simulink model "turbines2tune"  (R2025b)
settings: Solver=FixedStepAuto  StartTime=0.0  StopTime=200  FixedStep=Ts_outer  RelTol=1e-3
InitFcn:
  | turbine_model_constants;
values from neighbouring files (symbols this model uses):
  A = Simulink.Parameter(R.Value^2*pi)    [turbine_constants_from_yaml.m]    (also in turbine_model_constants.m)
  beta_opt_vector = Simulink.Parameter(beta_array)    [turbine_constants_from_yaml.m]    (also in turbine_model_constants.m)
  beta_vector = tables{4}    [gen_xref_ref.m]    (also in get_look_up_tables.m = zeros(1, 20); turbine_constants_from_yaml.m = Simulink.Parameter(tables{4}); turbine_model_constants.m = Simulink.Parameter(tables{4}))
  c_beta_dot = Simulink.Parameter(0.5)    [turbine_constants_from_yaml.m]    (also in turbine_model_constants.m = Simulink.Parameter(0.1))
  c_gamma_dot = Simulink.Parameter(0.5*pi/180)    [turbine_constants_from_yaml.m]    (also in turbine_model_constants.m = Simulink.Parameter(1/180*pi))
  cp_max = Simulink.Parameter(max(cp_table.Value(:))*0.99)    [turbine_constants_from_yaml.m]    (also in turbine_model_constants.m)
  cp_opt_keys = Simulink.Parameter(cell2mat(cp_vector))    [turbine_constants_from_yaml.m]    (also in turbine_model_constants.m)
  cp_table = tables{1}    [gen_xref_ref.m]    (also in get_look_up_tables.m = zeros(20, 20); turbine_constants_from_yaml.m = Simulink.Parameter(tables{1}); turbine_model_constants.m = Simulink.Parameter(tables{1}))
  ct_table = tables{2}    [gen_xref_ref.m]    (also in get_look_up_tables.m = zeros(20, 20); turbine_constants_from_yaml.m = Simulink.Parameter(tables{2}); turbine_model_constants.m = Simulink.Parameter(tables{2}))
  JT = Simulink.Parameter(10^9)    [turbine_constants_from_yaml.m]    (also in turbine_model_constants.m = Simulink.Parameter(2.052*10^8*3))
  lambda_opt_vector = Simulink.Parameter(lambda_array)    [turbine_constants_from_yaml.m]    (also in turbine_model_constants.m)
  lambda_vector = tables{5}    [gen_xref_ref.m]    (also in turbine_constants_from_yaml.m = Simulink.Parameter(tables{5}); turbine_model_constants.m = Simulink.Parameter(tables{5}))
  mu = Simulink.Parameter(0.95)    [turbine_constants_from_yaml.m]    (also in turbine_model_constants.m)
  Nt = Simulink.Parameter(10)    [turbine_constants_from_yaml.m]    (also in turbine_model_constants.m)
  omega_safety_increase = Simulink.Parameter(1.0)    [turbine_constants_from_yaml.m]    (also in turbine_model_constants.m = Simulink.Parameter(1.02))
  P_omega_dot = Simulink.Parameter(0.01)    [turbine_constants_from_yaml.m]    (also in turbine_model_constants.m = Simulink.Parameter(0.5))
  P_omega_dot_negative = Simulink.Parameter(0.05)    [turbine_model_constants.m]
  R = Simulink.Parameter(80)    [turbine_constants_from_yaml.m]    (also in turbine_model_constants.m = Simulink.Parameter(142); visualise.m = linspace(0.2, 0.7, nColors)')
  rho = Simulink.Parameter(1.225)    [turbine_constants_from_yaml.m]    (also in turbine_model_constants.m)
  Ts = Simulink.Parameter(1)    [turbine_constants_from_yaml.m]    (also in turbine_model_constants.m = Simulink.Parameter(0.1))
  Ts_inner = Simulink.Parameter(1)    [turbine_model_constants.m]
  x0 = Simulink.Parameter([0,0,0])    [turbine_constants_from_yaml.m]    (also in turbine_model_constants.m)
undefined symbols (not defined in the file or in its folder): DiscIntNeverNeededParam, f
libraries: instrumentlib x3, simulink_extras x1
settings Model: Creator=kohlh  LastModifiedBy=akohlheb

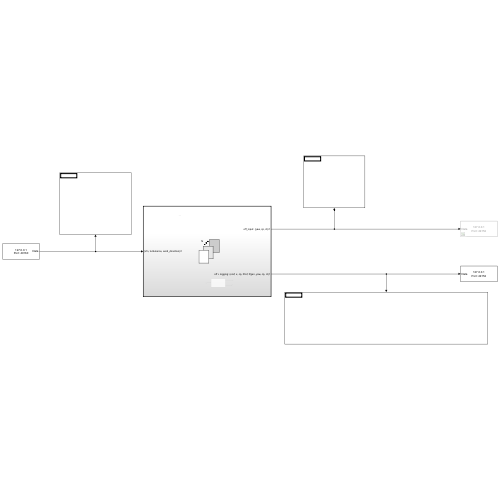
[thumbnail: Simulink's stored preview of the top-level diagram]
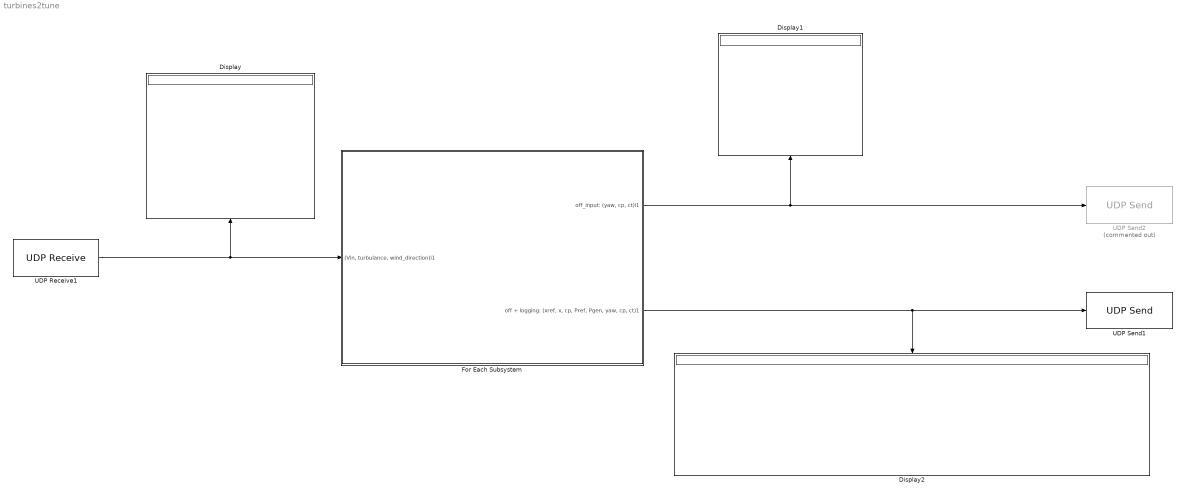
== system turbines2tune ==
  Display : Display
  Display1 : Display
  Display2 : Display
  For Each Subsystem : Subsystem  TreatAsAtomicUnit=on
  UDP Receive1 : instrumentlib/UDP Receive  LocalAddress=127.0.0.1  LocalPort=49160  EnablePortSharing=off  Host=127.0.0.1  Port=49152  GetLatestData=off  DataSize=[Nt,3]  DataType=double  ASCIIFormatting=%f,  Terminator=LF  CustomTerminator=10  ByteOrder=big-endian  EnableBlockingMode=on  Timeout=30  SampleTime=Ts  SimulateUsing=Interpreted execution
  UDP Send1 : instrumentlib/UDP Send  Host=127.0.0.1  Port=49152  LocalAddress=127.0.0.1  LocalPort=49160  EnablePortSharing=off  OutputDatagramPacketSize=512*12*Nt  ByteOrder=big-endian  EnableBlockingMode=on  SimulateUsing=Interpreted execution
  UDP Send2 : instrumentlib/UDP Send  Commented=on  Host=127.0.0.1  Port=49152  LocalAddress=127.0.0.1  LocalPort=49160  EnablePortSharing=off  OutputDatagramPacketSize=512*3*Nt  ByteOrder=big-endian  EnableBlockingMode=on  SimulateUsing=Interpreted execution
  wires:
  UDP Receive1/1 -> For Each Subsystem/1("(Vin, turbulance, wind_direction)i1"), Display/1
  For Each Subsystem/2("off + logging: (xref, x, cp, Pref, Pgen, yaw, cp, ct)1") -> UDP Send1/1, Display2/1
  For Each Subsystem/1("off_input: (yaw, cp, ct)i1") -> Display1/1, UDP Send2/1

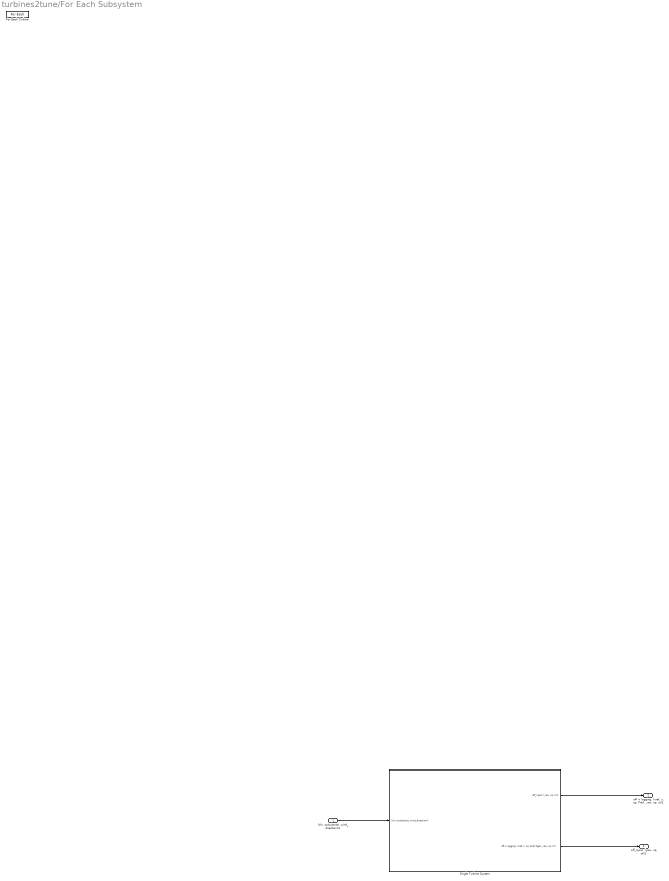
== system turbines2tune/For Each Subsystem ==
  "(Vin, turbulance, wind_direction)i1" : Inport  Partition=on  PartitionDimension=1  PartitionWidth=1  PartitionOffset=0
  For Each Turbine : ForEach  DisableCoverage=on
  Single Turbine System : Subsystem
  "off_input: (yaw, cp, ct)i1" : Outport  ConcatenationDimension=1
  "off + logging: (xref, x, cp, Pref, Pgen, yaw, cp, ct)1" : Outport  Port=2  ConcatenationDimension=1
  wires:
  "(Vin, turbulance, wind_direction)i1"/1 -> Single Turbine System/1("(Vin, turbulance, wind_direction)i")
  Single Turbine System/2("off + logging: (xref, x, cp, Pref, Pgen, yaw, cp, ct)") -> "off_input: (yaw, cp, ct)i1"/1
  Single Turbine System/1("off_input: (yaw, cp, ct)i") -> "off + logging: (xref, x, cp, Pref, Pgen, yaw, cp, ct)1"/1

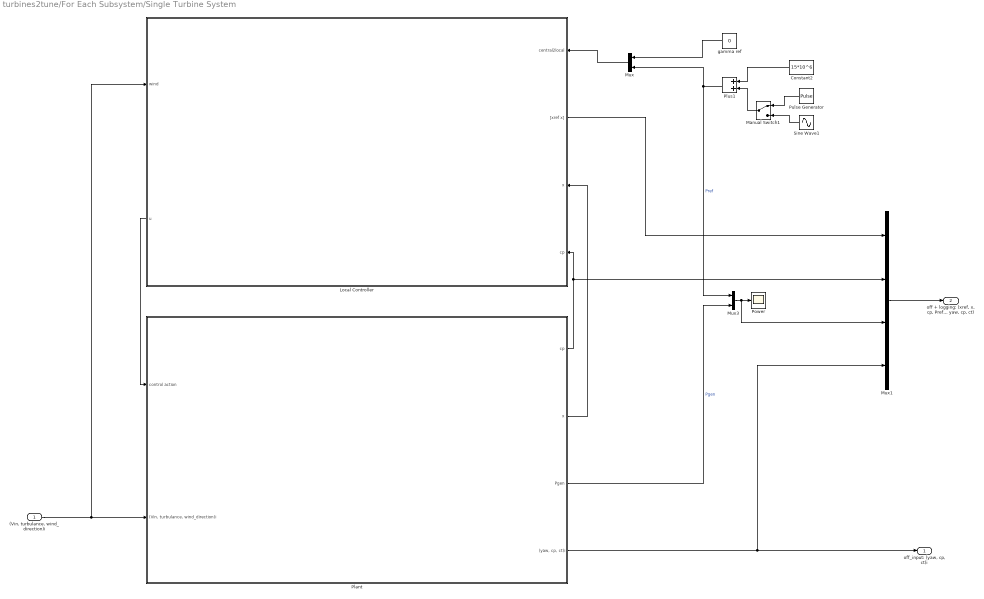
== system turbines2tune/For Each Subsystem/Single Turbine System ==
  "(Vin, turbulance, wind_direction)i" : Inport
  Constant2 : Constant  Value=15*10^6
  Local Controller : Subsystem
      settings: PortSchema="{\"entries\":[{\"content\":{\"sides\":[{\"content\":{\"connectorIds\":[\"In1\",\"Out2\",\"In2\",\"In3\"]},\"type\":\"ConnectorPlacement.EquallySpacedRectSide\",\"uuid\":\"1274bf49-ceae-40b5-8168-864c275c8277\"},{\"content\":{\"connectorIds\":[\"In4\",\"Out1\"],\"side\":\"RIGHT\"},\"type\":\"ConnectorPlacement.EquallySpacedRectSide\",\"uuid\":\"983d855e-2fb7-4029-8a1e-74d0395d6e6b\"},{\"content\":{\"side\":\"TOP\"},\"type\":\"ConnectorPlacement.EquallySpacedRectSide\",\"uuid\":\"78e40a3c-46aa-4158-bc61-97e5b88f823b\"},{\"content\":{\"side\":\"BOTTOM\"},\"type\":\"ConnectorPlacement.EquallySpacedRectSide\",\"uuid\":\"db79cd87-5583-4254-9385-067380eca232\"}]},\"type\":\"ConnectorPlacement.EquallySpacedConnector\",\"uuid\":\"902a270f-1fdc-458f-b9eb-4015978e6616\"}],\"packageUris\":[\"http://schema.mathworks.com/mf0/Connector/R2020b\"],\"version\":\"1.0\"}"
  Manual Switch1 : ManualSwitch
  Mux : Mux  Inputs=2
  Mux1 : Mux
  Mux3 : Mux  Inputs=2
  Plant : Subsystem
  Plus1 : Sum
  Power : Scope
      settings: ActiveDisplayYMinimum=-2.5E+6  ActiveDisplayYMaximum=2.2500000000000004E+7  DataLoggingVariableName=ScopeData2
  Pulse Generator : DiscretePulseGenerator  PulseType=Time based  Amplitude=5*10^6  Period=4000  PulseWidth=50
  Sine Wave1 : Sin  Amplitude=5*10^6  Frequency=3.24/1000  SampleTime=0
  gamma ref : Constant  Value=0
  "off_input: (yaw, cp, ct)i" : Outport
  "off + logging: (xref, x, cp, Pref, Pgen, yaw, cp, ct)" : Outport  Port=2
  wires:
  Local Controller/2("[xref x]") -> Mux1/1
  Plus1/1 -> Mux/2, Mux3/1  "Pref"
  Constant2/1 -> Plus1/1
  Manual Switch1/1 -> Plus1/2
  Mux/1 -> Local Controller/1(central2local)
  Pulse Generator/1 -> Manual Switch1/1
  Plant/3(Pgen) -> Mux3/2  "Pgen"
  "(Vin, turbulance, wind_direction)i"/1 -> Local Controller/4(wind), Plant/2("(Vin, turbulance, wind_direction)i")
  Mux1/1 -> "off + logging: (xref, x, cp, Pref, Pgen, yaw, cp, ct)"/1
  Sine Wave1/1 -> Manual Switch1/2
  Local Controller/1(u) -> Plant/1(control action)
  Plant/4("(yaw, cp, ct)i") -> Mux1/4, "off_input: (yaw, cp, ct)i"/1
  Plant/1(cp) -> Local Controller/3(cp), Mux1/2
  Plant/2(x) -> Local Controller/2(x)
  Mux3/1 -> Mux1/3, Power/1
  gamma ref/1 -> Mux/1

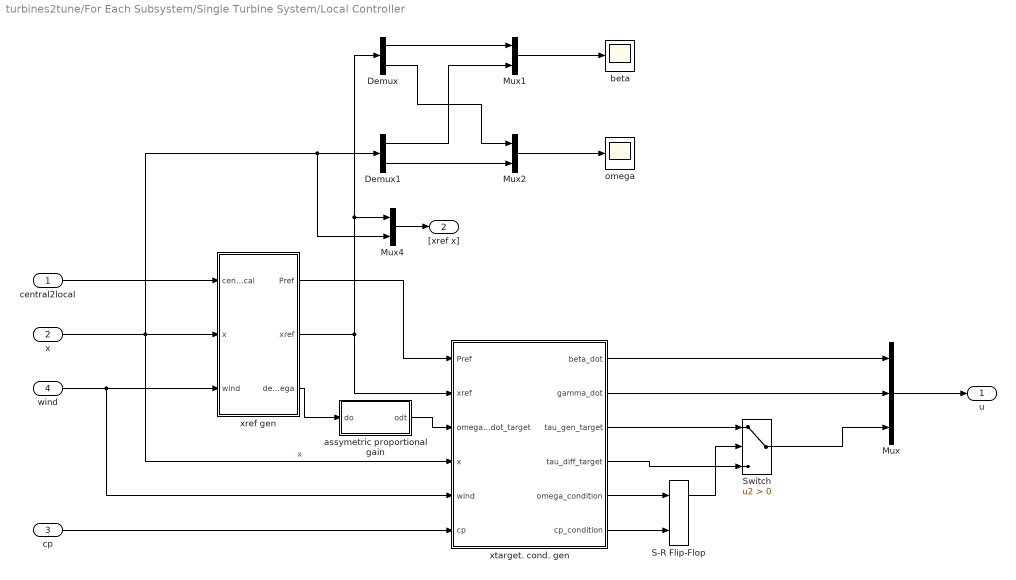
== system turbines2tune/For Each Subsystem/Single Turbine System/Local Controller ==
  central2local : Inport
  x : Inport  Port=2
  cp : Inport  Port=3
  wind : Inport  Port=4
  Demux : Demux  Outputs=3
  Demux1 : Demux  Outputs=3
  Mux : Mux  Inputs=3
  Mux1 : Mux  Inputs=2
  Mux2 : Mux  Inputs=2
  Mux4 : Mux  Inputs=2
  S-R Flip-Flop : simulink_extras/Flip Flops/S-R Flip-Flop  initial_condition=0
  Switch : Switch  Criteria=u2 > Threshold  SaturateOnIntegerOverflow=off  InputSameDT=off
  assymetric proportional gain : MATLAB Function  TreatAsAtomicUnit=on
  beta : Scope
      settings: ActiveDisplayYMinimum=-2.9999999999999991  ActiveDisplayYMaximum=27
  omega : Scope
      settings: ActiveDisplayYMinimum=-0.25747285201612957  ActiveDisplayYMaximum=2.3172556681451666
  xref gen : MATLAB Function  TreatAsAtomicUnit=on
  xtarget. cond. gen : MATLAB Function  TreatAsAtomicUnit=on
  u : Outport
  "[xref x]" : Outport  Port=2
  wires:
  central2local/1 -> xref gen/1(central2local)
  xref gen/2(xref) -> Mux4/1, Demux/1, xtarget. cond. gen/2(xref)
  Mux/1 -> u/1
  xtarget. cond. gen/1(beta_dot) -> Mux/1
  xtarget. cond. gen/2(gamma_dot) -> Mux/2
  xtarget. cond. gen/3(tau_gen_target) -> Switch/1
  xtarget. cond. gen/4(tau_diff_target) -> Switch/3
  xtarget. cond. gen/6(cp_condition) -> S-R Flip-Flop/2
  x/1 -> xtarget. cond. gen/4(x), Mux4/2, Demux1/1, xref gen/2(x)  "x"
  wind/1 -> xtarget. cond. gen/5(wind), xref gen/3(wind)
  Switch/1 -> Mux/3
  S-R Flip-Flop/1 -> Switch/2
  xtarget. cond. gen/5(omega_condition) -> S-R Flip-Flop/1
  cp/1 -> xtarget. cond. gen/6(cp)
  xref gen/3(delta_omega) -> assymetric proportional gain/1(do)
  xref gen/1(Pref) -> xtarget. cond. gen/1(Pref)
  Mux1/1 -> beta/1
  Mux2/1 -> omega/1
  Demux/1 -> Mux1/1
  Demux1/3 -> Mux2/2
  Demux1/1 -> Mux1/2
  Demux/3 -> Mux2/1
  Mux4/1 -> "[xref x]"/1
  assymetric proportional gain/1(odt) -> xtarget. cond. gen/3(omega_dot_target)

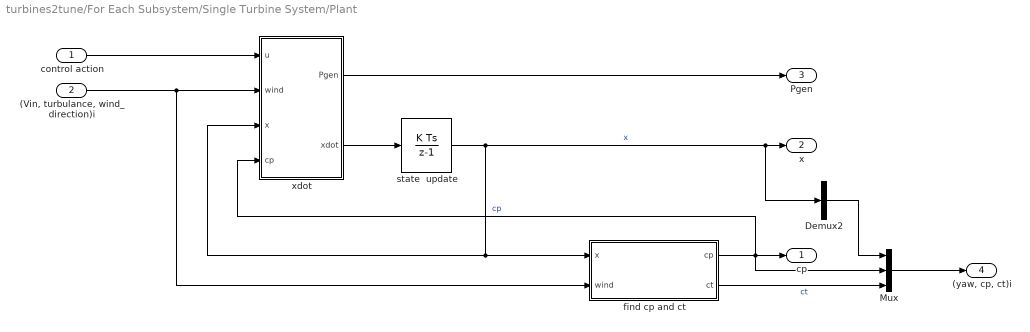
== system turbines2tune/For Each Subsystem/Single Turbine System/Plant ==
  control action : Inport
  "(Vin, turbulance, wind_direction)i" : Inport  Port=2
  Demux2 : Demux  Outputs=3
  Mux : Mux  Inputs=3
  find cp and ct : MATLAB Function  TreatAsAtomicUnit=on
  state  update : DiscreteIntegrator  InitialCondition=x0  SampleTime=-1  LimitOutput=on  ICPrevOutput=DiscIntNeverNeededParam  ICPrevScaledInput=DiscIntNeverNeededParam
  xdot : MATLAB Function  TreatAsAtomicUnit=on
  cp : Outport
  x : Outport  Port=2
  Pgen : Outport  Port=3
  "(yaw, cp, ct)i" : Outport  Port=4
  wires:
  "(Vin, turbulance, wind_direction)i"/1 -> find cp and ct/2(wind), xdot/2(wind)
  xdot/2(xdot) -> state  update/1
  state  update/1 -> Demux2/1, x/1, find cp and ct/1(x), xdot/3(x)  "x"
  control action/1 -> xdot/1(u)
  xdot/1(Pgen) -> Pgen/1
  find cp and ct/1(cp) -> Mux/2, cp/1, xdot/4(cp)  "cp"
  find cp and ct/2(ct) -> Mux/3  "ct"
  Demux2/2 -> Mux/1
  Mux/1 -> "(yaw, cp, ct)i"/1

== matlab function turbines2tune/For Each Subsystem/Single Turbine System/Plant/xdot ==
  data: Pgen output; u input; xdot output; wind input; x input; cp input; JT parameter; A parameter; rho parameter; mu parameter
function [Pgen, xdot] = fcn(u, wind, x, cp, JT, A, rho, mu)

Vin = wind(1);
turbulance = 1-wind(2);
wind_direction = wind(3);

beta_dot = u(1);
gamma_dot = u(2);
tau_gen = u(3);

gamma = x(2);
omega = x(3);

%eliminating division by 0
if omega < 0.1 && omega >= 0
    omega = 0.1;
    tau_gen = 0;
    % if there is no motion backwards acc due to tau aero is not allowed
    tau_aero = max(0, cp * Vin^3 * rho * A * 1/2 * turbulance * cos(wind_direction-gamma)^3 / omega);
elseif omega < 0
    tau_aero = abs(cp * Vin^3 * rho * A * 1/2 * turbulance * cos(wind_direction-gamma)^3 / omega);
    tau_gen = 0;
else
    tau_aero = cp * Vin^3 * rho * A * 1/2 * turbulance * cos(wind_direction-gamma)^3 / omega;
end

omega_dot = (tau_aero - tau_gen)/JT;

xdot = [beta_dot, gamma_dot, omega_dot];
Pgen = tau_gen * omega * mu;

end

== matlab function turbines2tune/For Each Subsystem/Single Turbine System/Local Controller/assymetric proportional gain ==
  data: do input; odt output; P_omega_dot parameter; P_omega_dot_negative parameter
function odt = P(do, P_omega_dot, P_omega_dot_negative)
if do > 0
    odt = P_omega_dot * do;
else
    odt = P_omega_dot_negative * do;
end

== matlab function turbines2tune/For Each Subsystem/Single Turbine System/Local Controller/xref gen ==
  data: central2local input; Pref output; x input; wind input; xref output; mu parameter; lambda_vector parameter; beta_vector parameter; cp_table parameter; R parameter; rho parameter; A parameter; cp_max parameter; delta_omega output; cp_opt_keys parameter; beta_opt_vector parameter; c_beta_dot parameter; Ts_inner parameter; lambda_opt_vector parameter
function [Pref, xref, delta_omega] = xrefgen(central2local,  x, wind, mu, lambda_vector, beta_vector, cp_table, R, rho, A, cp_max, cp_opt_keys, beta_opt_vector, c_beta_dot, Ts_inner, lambda_opt_vector)
    Vin = wind(1);
    turbulance = 1-wind(2);
    wind_direction = wind(3);

    Pref = central2local(2);
    gamma_ref = wind_direction; %central2local(1);
    
    beta = x(1);
    gamma = x(2);
    omega = x(3);
    
    %cap cpref to avoid oscillation at the boundary
    Pref = max(min(Pref, (1/2 * Vin^3 * rho * A * mu * turbulance*cos(wind_direction - gamma)^3)*cp_max),0);
    if cos(wind_direction - gamma) > 0
        cpref = Pref/(1/2 * Vin^3 * rho * A * mu * turbulance*cos(wind_direction - gamma)^3);
    else
        cpref = 0;
    end

    
    %find closest cp opt key that is larger than cpref
    [closest_cp, ~] = min(abs((cp_opt_keys >= cpref) - cpref));
    [~,closest_cp_index] = min(abs(cp_opt_keys - closest_cp));
    beta_opt = beta_opt_vector(closest_cp_index);
    %find beta that is achieveable with delta beta due to descrete steps
    deltabeta = c_beta_dot * Ts_inner;
    beta_over = ceil((beta_opt - beta)/deltabeta) * deltabeta + beta;
    beta_under = floor((beta_opt - beta)/deltabeta) * deltabeta + beta;

    beta_ref = beta_under;

    cp_at_beta_opt = NaN;
    for i = 1:length(beta_vector)-1
        if beta_vector(i) <= beta_ref && beta_vector(i+1) >= beta_ref
            cp_at_beta_opt = cp_table(1:end,i) * abs((beta_ref - beta_vector(i+1))/(beta_vector(i+1) - beta_vector(i))) + cp_table(1:end,i+1) * abs((beta_ref - beta_vector(i))/(beta_vector(i+1) - beta_vector(i)));
            break
        end
    end

    lambda_ref = NaN;
    for i = 1:length(beta_vector)-1
        if (cp_at_beta_opt(i) <= cpref && cp_at_beta_opt(i+1) >= cpref) || (cp_at_beta_opt(i+1) <= cpref && cp_at_beta_opt(i) >= cpref)
            lambda_ref = lambda_vector(i) * abs((cpref - cp_at_beta_opt(i+1))/(cp_at_beta_opt(i+1) - cp_at_beta_opt(i))) + lambda_vector(i+1) * abs((cpref - cp_at_beta_opt(i))/(cp_at_beta_opt(i+1) - cp_at_beta_opt(i)));
            break
        end
    end

    if isnan(lambda_ref)
        beta_ref = beta_over;

        for i = 1:length(beta_vector)-1
            if beta_vector(i) <= beta_ref && beta_vector(i+1) >= beta_ref
                cp_at_beta_opt = cp_table(1:end,i) * abs((beta_ref - beta_vector(i+1))/(beta_vector(i+1) - beta_vector(i))) + cp_table(1:end,i+1) * abs((beta_ref - beta_vector(i))/(beta_vector(i+1) - beta_vector(i)));
                break
            end
        end

        for i = 1:length(beta_vector)-1
            if (cp_at_beta_opt(i) <= cpref && cp_at_beta_opt(i+1) >= cpref) || (cp_at_beta_opt(i+1) <= cpref && cp_at_beta_opt(i) >= cpref)
                lambda_ref = lambda_vector(i) * abs((cpref - cp_at_beta_opt(i+1))/(cp_at_beta_opt(i+1) - cp_at_beta_opt(i))) + lambda_vector(i+1) * abs((cpref - cp_at_beta_opt(i))/(cp_at_beta_opt(i+1) - cp_at_beta_opt(i)));
                break
            end
        end
    end
    if isnan(lambda_ref)
        beta_ref = beta_opt;
        for i = 1:length(beta_vector)-1
            if beta_vector(i) <= beta_ref && beta_vector(i+1) >= beta_ref
                cp_at_beta_opt = cp_table(1:end,i) * abs((beta_ref - beta_vector(i+1))/(beta_vector(i+1) - beta_vector(i))) + cp_table(1:end,i+1) * abs((beta_ref - beta_vector(i))/(beta_vector(i+1) - beta_vector(i)));
                break
            end
        end

        for i = 1:length(beta_vector)-1
            if (cp_at_beta_opt(i) <= cpref && cp_at_beta_opt(i+1) >= cpref) || (cp_at_beta_opt(i+1) <= cpref && cp_at_beta_opt(i) >= cpref)
                lambda_ref = lambda_vector(i) * abs((cpref - cp_at_beta_opt(i+1))/(cp_at_beta_opt(i+1) - cp_at_beta_opt(i))) + lambda_vector(i+1) * abs((cpref - cp_at_beta_opt(i))/(cp_at_beta_opt(i+1) - cp_at_beta_opt(i)));
                break
            end
        end
    end
    if isnan(lambda_ref)
        lambda_ref = lambda_opt_vector(closest_cp_index);
    end
    
    omega_ref = lambda_ref * Vin * cos(wind_direction - gamma) / R;   
    xref = [beta_ref, gamma_ref, omega_ref];
    delta_omega = (omega_ref - omega)/omega_ref;
end

== matlab function turbines2tune/For Each Subsystem/Single Turbine System/Local Controller/xtarget. cond. gen ==
  data: Pref input; xref input; omega_dot_target input; beta_dot output; gamma_dot output; tau_gen_target output; tau_diff_target output; omega_condition output; x input; wind input; cp input; R parameter; lambda_vector parameter; beta_vector parameter; cp_table parameter; mu parameter; rho parameter; A parameter; omega_safety_increase parameter; cp_condition output; Ts_inner parameter; c_beta_dot parameter; c_gamma_dot parameter; JT parameter
function [beta_dot, gamma_dot, tau_gen_target, tau_diff_target, omega_condition, cp_condition] = tg(Pref, xref,omega_dot_target, x, wind, cp, R, lambda_vector, beta_vector, cp_table, mu, rho, A, omega_safety_increase, Ts_inner, c_beta_dot, c_gamma_dot, JT)
beta = x(1);
gamma = x(2);
omega = x(3);

Vin = wind(1);
turbulance = 1-wind(2);
wind_direction = wind(3);

betaref = xref(1);
gammaref = xref(2);
omegaref = xref(3);

lambda = omega * R / (Vin * cos(wind_direction - gamma));

lambda_index_under = 0;
for i=1:length(lambda_vector)-1
    if lambda>lambda_vector(i)
        lambda_index_under = i;
    end
end

if lambda_index_under == 0
    lambda_under_coef = 1;
    lambda_index_under = 1;
elseif lambda > lambda_vector(end)
    lambda_under_coef = 0;
else
    lambda_under_coef = abs((lambda_vector(lambda_index_under+1) - lambda)/(lambda_vector(lambda_index_under) - lambda_vector(lambda_index_under+1)));
end

cp_at_omega = cp_table(lambda_index_under, 1:end) * lambda_under_coef +  cp_table(lambda_index_under+1, 1:end) * (1-lambda_under_coef);

if omega <= 0
    tau_gen_target = 0;
else
    tau_gen_target = Pref/(omega*mu);
end
if isnan(tau_gen_target)
    tau_gen_target = 0;
end

tau_aero_target = JT * omega_dot_target + tau_gen_target; % to reach omega dot target
if cos(wind_direction - gamma) > 0
    if omega > 0
        cp_target = tau_aero_target* omega / (1/2 * rho * A * Vin^3 * turbulance * cos(wind_direction - gamma)^3);
    elseif omega == 0
        cp_target = 0.5;
    else
        cp_target = -tau_aero_target* omega / (1/2 * rho * A * Vin^3 * turbulance * cos(wind_direction - gamma)^3);
    end
else
    cp_target = 0;
end

cpmin = abs(tau_gen_target * omega / (1/2 * rho * A * Vin^3 * turbulance * cos(wind_direction - gamma)^3));

cp_increase_direction = 1;
cp_target = max(0, cp_target);
if cp_target > max(cp_at_omega)
    [~, beta_upper_index] = max(cp_at_omega);
    beta_target_online = beta_vector(beta_upper_index);
else
    beta_target_online = nan;
    for i=length(beta_vector):-1:2 % going from higher beta valeus
        if (cp_at_omega(i-1) >= cp_target && cp_at_omega(i) <= cp_target) || (cp_at_omega(i) >= cp_target && cp_at_omega(i-1) <= cp_target)
            beta_target_upper_index = i;
            beta_upper_coef = abs((cp_at_omega(beta_target_upper_index-1)- cp_target)/(cp_at_omega(beta_target_upper_index-1) - cp_at_omega(beta_target_upper_index)));
            beta_target_online = beta_vector(beta_target_upper_index) * beta_upper_coef + beta_vector(beta_target_upper_index-1) * (1-beta_upper_coef);
            if cp_at_omega(i-1) <= cp_at_omega(i)
                cp_increase_direction = 1;
            else
                cp_increase_direction = -1;
            end
            break
        end
    end
end

beta_target = beta_target_online;

if abs(beta_target - beta) > Ts_inner * c_beta_dot
    if beta_target > beta
        beta_dot = c_beta_dot;
    else
        beta_dot = -c_beta_dot;
    end
else
    if abs(omega_dot_target) > 10^(-5)
        if omega_dot_target > 0
            if beta_target > beta
                if cp_increase_direction > 0
                    beta_dot = c_beta_dot;
                else
                    beta_dot = 0;
                end
            else
                if cp_increase_direction > 0
                    beta_dot = 0;
                else
                    beta_dot = -c_beta_dot;
                end
            end
        elseif omega_dot_target < 0
            if beta_target > beta
                if cp_increase_direction > 0
                    beta_dot = 0;
                else
                    beta_dot = c_beta_dot;
                end
            else
                if cp_increase_direction > 0
                    beta_dot = -c_beta_dot;
                else
                    beta_dot = 0;
                end
            end
        else
            beta_dot = 0;
        end
    else
        if abs(betaref - beta) > Ts_inner * c_beta_dot * 0.5
            if betaref > beta
                beta_dot = c_beta_dot;
            else
                beta_dot = -c_beta_dot;
            end
        else
            beta_dot = 0;
        end
    end
end



if abs(gammaref - gamma) > Ts_inner * c_gamma_dot * 0.5
    if gammaref > gamma
        gamma_dot = c_gamma_dot;
    else
        gamma_dot = -c_gamma_dot;
    end
else
    gamma_dot = 0;
end


if cpmin > max(cp_at_omega) && omega < omegaref*omega_safety_increase
    omega_condition = false;
    cp_condition = true;
elseif omega >= omegaref * omega_safety_increase
    omega_condition = true;
    cp_condition = false;
else
    omega_condition = false;
    cp_condition = false;
end
if omega <= 0
    tau_diff_target = 0;
else
    tau_diff_target = min(max(cp*(1/2 * rho * A * Vin^3 * turbulance * cos(wind_direction - gamma)^3)/omega - JT * omega_dot_target), tau_gen_target);
end

end

== matlab function turbines2tune/For Each Subsystem/Single Turbine System/Plant/find cp and ct ==
  data: x input; cp output; ct output; wind input; R parameter; beta_vector parameter; lambda_vector parameter; cp_table parameter; ct_table parameter
function [cp, ct] = lookup(x, wind, R, beta_vector, lambda_vector, cp_table, ct_table)
beta = x(1);
gamma = x(2);
omega = x(3);

Vin = wind(1);
wind_direction = wind(3);

lambda = omega * R/ (Vin * cos(wind_direction - gamma));

beta_index_under = 0;
for i=1:length(beta_vector)-1
    if beta>beta_vector(i)
        beta_index_under = i;
    end
end

lambda_index_under = 0;
for i=1:length(lambda_vector)-1
    if lambda>lambda_vector(i)
        lambda_index_under = i;
    end
end

if beta_index_under == 0
    beta_under_coef = 1;
    beta_index_under = 1;
elseif beta > beta_vector(end)
    beta_under_coef = 0;
else
    beta_under_coef = abs((beta_vector(beta_index_under+1) - beta)/(beta_vector(beta_index_under) - beta_vector(beta_index_under+1)));
end

if lambda_index_under == 0
    lambda_under_coef = 1;
    lambda_index_under = 1;
elseif lambda > lambda_vector(end)
    lambda_under_coef = 0;
else
    lambda_under_coef = abs((lambda_vector(lambda_index_under+1) - lambda)/(lambda_vector(lambda_index_under) - lambda_vector(lambda_index_under+1)));
end

cp = cp_table(lambda_index_under, beta_index_under) * (beta_under_coef * lambda_under_coef) ...
    + cp_table(lambda_index_under+1, beta_index_under) * ((1 - lambda_under_coef) * beta_under_coef) ...
    + cp_table(lambda_index_under, beta_index_under+1) * (lambda_under_coef * (1 - beta_under_coef)) ...
    + cp_table(lambda_index_under+1, beta_index_under+1) * ((1 - lambda_under_coef) * (1 - beta_under_coef));

ct = ct_table(lambda_index_under, beta_index_under) * (beta_under_coef * lambda_under_coef) ...
    + ct_table(lambda_index_under+1, beta_index_under) * ((1 - lambda_under_coef) * beta_under_coef) ...
    + ct_table(lambda_index_under, beta_index_under+1) * (lambda_under_coef * (1 - beta_under_coef)) ...
    + ct_table(lambda_index_under+1, beta_index_under+1) * ((1 - lambda_under_coef) * (1 - beta_under_coef));
end
